simulink model "Es6_sim"  (R2018b)
settings: Solver=VariableStepAuto  StartTime=0.0  StopTime=10.0  RelTol=1e-3
libraries: simulink x1
settings Model: Creator=utente  LastModifiedBy=utente

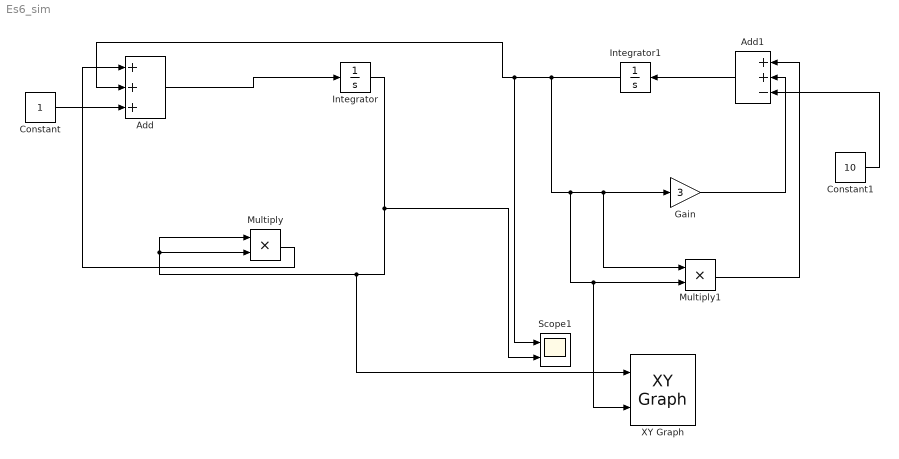
== system Es6_sim ==
  Add : Sum  Inputs=+++
  Add1 : Sum  Inputs=++-
  Constant : Constant
  Constant1 : Constant  Value=10
  Gain : Gain  Gain=3
  Integrator : Integrator  InitialCondition=-5
  Integrator1 : Integrator
  Multiply : Product
  Multiply1 : Product
  Scope1 : Scope  NumInputPorts=2
  XY Graph : simulink/Sinks/XY Graph  xmin=-10  xmax=10  ymin=-10  ymax=10  st=1
  wires:
  Integrator1/1 -> XY Graph/2, Multiply1/2, Multiply1/1, Gain/1, Scope1/1, Add/2
  Constant/1 -> Add/3
  Add1/1 -> Integrator1/1
  Gain/1 -> Add1/2
  Constant1/1 -> Add1/3
  Integrator/1 -> Scope1/2, XY Graph/1, Multiply/2, Multiply/1
  Multiply/1 -> Add/1
  Multiply1/1 -> Add1/1
  Add/1 -> Integrator/1
